simulink model "ABS_system"  (R2020b)
settings: Solver=VariableStepAuto  StartTime=0.0  StopTime=20  RelTol=1e-3
InitFcn:
  | m = 75;   % mass of vehicle
  | g = 9.81; % gravitational constant
  | I = 5;    % moment of inertia
  | R = 1.25; % radius of wheel
  | v0 = 44;  % initial vehicle speed
  | 
  | open_system("ABS_system/Wheel&VehicleSpeed");
  | open_system("ABS_system/VehicleSlip");
  | open_system("ABS_system/StoppingDistance");
settings Model: Creator=sneha  LastModifiedBy=sneha

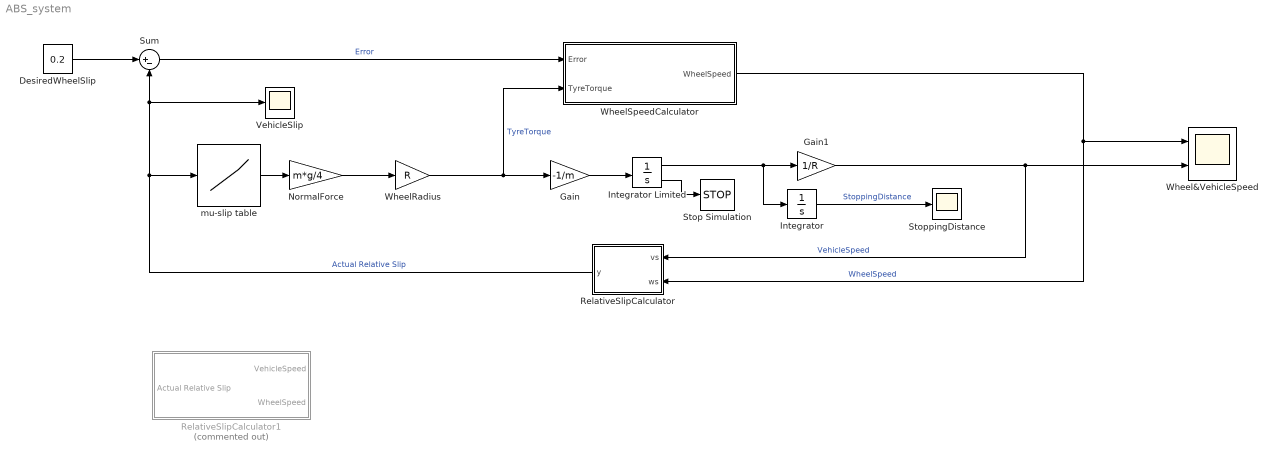
== system ABS_system ==
  "\tRelativeSlipCalculator" : MATLAB Function  TreatAsAtomicUnit=on
  DesiredWheelSlip : Constant  Value=0.2
  Gain : Gain  Gain=-1/m
  Gain1 : Gain  Gain=1/R
  Integrator : Integrator
  Integrator Limited : Integrator  InitialCondition=v0  LimitOutput=on  UpperSaturationLimit=1000  LowerSaturationLimit=0  ShowSaturationPort=on
  NormalForce : Gain  Gain=m*g/4
  RelativeSlipCalculator1 : Subsystem  Commented=on
  Stop Simulation : Stop
  StoppingDistance : Scope
  Sum : Sum  Inputs=|+-
  VehicleSlip : Scope
  Wheel&VehicleSpeed : Scope  NumInputPorts=2
  WheelRadius : Gain  Gain=R
  WheelSpeedCalculator : Subsystem
  mu-slip table : Lookup_n-D  NumberOfTableDimensions=1  BreakpointsForDimension1=|  Table=|  InternalRulePriority=Speed  RndMeth=Simplest  InputSameDT=on
      BreakpointsForDimension1=|
      | [0
      | ,0.05
      | ,0.1
      | ,0.15
      | ,0.2
      | ,0.25
      | ,0.3
      | ,0.35
      | ,0.4
      | ,0.45
      | ,0.5
      | ,0.55
      | ,0.6
      | ,0.65
      | ,0.7
      | ,0.75
      | ,0.8
      | ,0.85
      | ,0.9
      | ,0.95
      | ,1]
      Table=|
      | [0
      | ,0.4
      | ,0.8
      | ,0.97
      | ,1
      | ,0.98
      | ,0.96
      | ,0.94
      | ,0.92
      | ,0.9
      | ,0.88
      | ,0.855
      | ,0.83
      | ,0.81
      | ,0.79
      | ,0.77
      | ,0.75
      | ,0.73
      | ,0.72
      | ,0.71
      | ,0.7]
  wires:
  DesiredWheelSlip/1 -> Sum/1
  mu-slip table/1 -> NormalForce/1
  NormalForce/1 -> WheelRadius/1
  Sum/1 -> WheelSpeedCalculator/1(Error)  "Error"
  WheelRadius/1 -> Gain/1, WheelSpeedCalculator/2(TyreTorque)  "TyreTorque"
  WheelSpeedCalculator/1(WheelSpeed) -> "\tRelativeSlipCalculator"/2(ws), Wheel&VehicleSpeed/1  "WheelSpeed"
  Gain/1 -> Integrator Limited/1
  Integrator Limited/1 -> Integrator/1, Gain1/1
  Gain1/1 -> "\tRelativeSlipCalculator"/1(vs), Wheel&VehicleSpeed/2  "VehicleSpeed"
  Integrator Limited/2 -> Stop Simulation/1
  Integrator/1 -> StoppingDistance/1  "StoppingDistance"
  "\tRelativeSlipCalculator"/1(y) -> mu-slip table/1, Sum/2, VehicleSlip/1  "Actual Relative Slip"

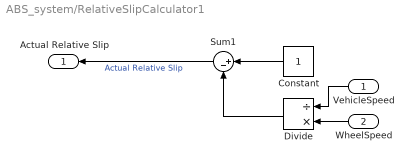
== system ABS_system/RelativeSlipCalculator1 ==
  VehicleSpeed : Inport
  WheelSpeed : Inport  Port=2
  Constant : Constant
  Divide : Product  Inputs=/*
  Sum1 : Sum  Inputs=|+-
  Actual Relative Slip : Outport
  wires:
  VehicleSpeed/1 -> Divide/1
  WheelSpeed/1 -> Divide/2
  Sum1/1 -> Actual Relative Slip/1  "Actual Relative Slip"
  Divide/1 -> Sum1/2
  Constant/1 -> Sum1/1

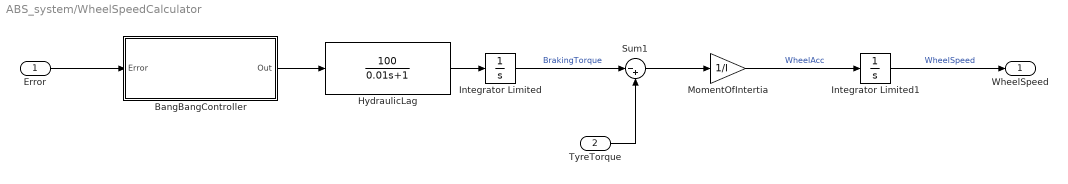
== system ABS_system/WheelSpeedCalculator ==
  Error : Inport
  TyreTorque : Inport  Port=2
  BangBangController : Subsystem
  HydraulicLag : TransferFcn  Numerator=[100]  Denominator=[0.01 1]
  Integrator Limited : Integrator  LimitOutput=on  UpperSaturationLimit=1000  LowerSaturationLimit=0
  Integrator Limited1 : Integrator  InitialCondition=v0/R  LimitOutput=on  UpperSaturationLimit=1000  LowerSaturationLimit=0
  MomentOfIntertia : Gain  Gain=1/I
  Sum1 : Sum  Inputs=|-+
  WheelSpeed : Outport
  wires:
  Sum1/1 -> MomentOfIntertia/1
  BangBangController/1(Out) -> HydraulicLag/1
  Error/1 -> BangBangController/1(Error)
  HydraulicLag/1 -> Integrator Limited/1
  TyreTorque/1 -> Sum1/2
  Integrator Limited/1 -> Sum1/1  "BrakingTorque"
  Integrator Limited1/1 -> WheelSpeed/1  "WheelSpeed"
  MomentOfIntertia/1 -> Integrator Limited1/1  "WheelAcc"

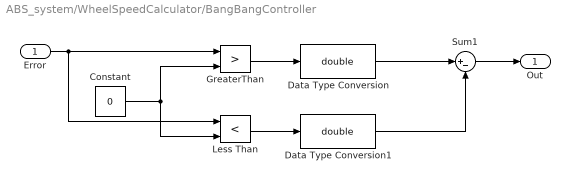
== system ABS_system/WheelSpeedCalculator/BangBangController ==
  Error : Inport
  Constant : Constant  Value=0
  Data Type Conversion : DataTypeConversion  OutDataTypeStr=double  RndMeth=Zero
  Data Type Conversion1 : DataTypeConversion  OutDataTypeStr=double  RndMeth=Zero
  GreaterThan : RelationalOperator  Operator=>  OutDataTypeStr=boolean  RndMeth=Simplest
  Less Than : RelationalOperator  Operator=<  OutDataTypeStr=boolean  RndMeth=Simplest
  Sum1 : Sum  Inputs=|+-
  Out : Outport
  wires:
  GreaterThan/1 -> Data Type Conversion/1
  Data Type Conversion/1 -> Sum1/1
  Constant/1 -> Less Than/2, GreaterThan/2
  Error/1 -> Less Than/1, GreaterThan/1
  Data Type Conversion1/1 -> Sum1/2
  Less Than/1 -> Data Type Conversion1/1
  Sum1/1 -> Out/1

== matlab function ABS_system/	RelativeSlipCalculator ==
  data: vs input; y output; ws input
function y = fcn(vs,ws)
y = 1-(ws/vs);
